simulink library "sensor_library"  (R2018b)
settings: Solver=VariableStepAuto  StartTime=0.0  StopTime=10.0  RelTol=1e-3
undefined symbols (not defined in the file): DiscIntNeverNeededParam, EOP_IERS, GPS, GPS_sensor_time, GYRO, GYRO_sensor_time, jdate0
libraries: dspsigops x26, simulink x9, simulink_extras x4
(part 1 of 2)
settings Model: Creator=Andrea  LastModifiedBy=andrea

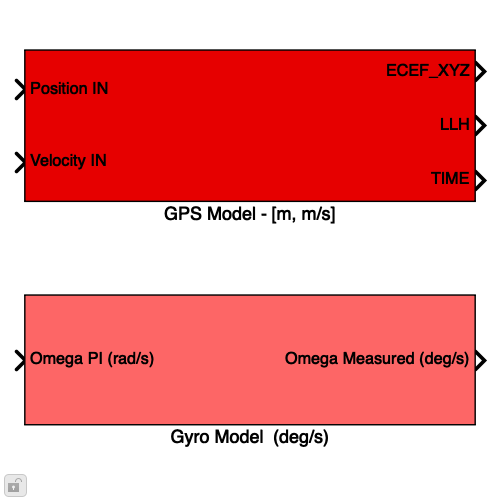
[thumbnail: Simulink's stored preview of the top-level diagram]
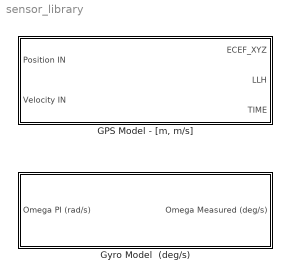
== system sensor_library ==
  "GPS Model - [m, m/s]" : Subsystem  mask{GPS=GPS, eop=EOP_IERS, jdutc_0=jdate0, simstep=GPS_sensor_time}
      mask prompts: GPS "GPS Data Structure"; eop "EOP (IERS) Parameter Structure"; jdutc_0 "Initial Simulation Time (UTC jdate)"; simstep "Sensor Time (s)"
  Gyro Model  (deg/s) : Subsystem  mask{gyros=GYRO.gyros, simstep=GYRO_sensor_time}
      mask prompts: gyros "Gyro Data Structure"; simstep "Sensor Time (s)"
      mask help:
      | Gyro Model - version A
      | Input - rad/s
      | Output - deg/s
      | Internal Data - deg/s

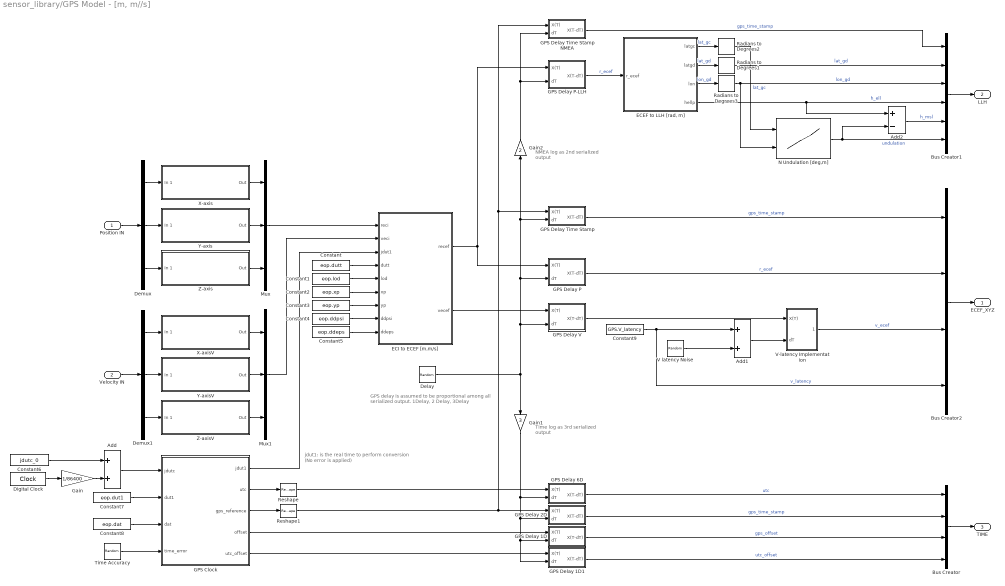
== system sensor_library/GPS Model - [m, m//s] ==
  note: NMEA log as 2nd
      | serialized output
  note: jdut1: is the real time to perform conversion
      | (No error is applied)
  note: GPS delay is assumed to be proportional among
      | all serialized output. 1Delay, 2 Delay, 3Delay
  note: Time log as 3rd
      | serialized output
  Position IN : Inport
  Velocity IN : Inport  Port=2
  Add : Sum
  Add1 : Sum
  Add2 : Sum  Inputs=+-
  Bus Creator : BusCreator  Inputs=4
  Bus Creator1 : BusCreator  Inputs=6
  Bus Creator2 : BusCreator  Inputs=4
  Constant : Constant  Value=eop.dutt  SampleTime=GPS.sampletime
  Constant1 : Constant  Value=eop.lod  SampleTime=GPS.sampletime
  Constant2 : Constant  Value=eop.xp  SampleTime=GPS.sampletime
  Constant3 : Constant  Value=eop.yp  SampleTime=GPS.sampletime
  Constant4 : Constant  Value=eop.ddpsi  SampleTime=GPS.sampletime
  Constant5 : Constant  Value=eop.ddeps  SampleTime=GPS.sampletime
  Constant6 : Constant  Value=jdutc_0  SampleTime=GPS.sampletime
  Constant7 : Constant  Value=eop.dut1  SampleTime=GPS.sampletime
  Constant8 : Constant  Value=eop.dat  SampleTime=GPS.sampletime
  Constant9 : Constant  Value=GPS.V_latency  SampleTime=GPS.sampletime
  Delay : RandomNumber  Mean=GPS.delay  Variance=GPS.delay_noise^2  Seed=GPS.noiseseedT-50  SampleTime=GPS.sampletime
  Demux : Demux  Outputs=3
  Demux1 : Demux  Outputs=3
  Digital Clock : DigitalClock  SampleTime=GPS.sampletime
  "ECEF to LLH [rad, m]" : MATLAB Function  TreatAsAtomicUnit=on
  ECI to ECEF [m,m/s] : MATLAB Function  TreatAsAtomicUnit=on
  GPS Clock : MATLAB Function  TreatAsAtomicUnit=on
  GPS Delay 1D : Subsystem  mask(Discrete Time Delay){maxT=1, Ts=GPS.sampletime}
      mask prompts: maxT "Max Delay Time (s)"; Ts "Sample Time (s)"
      mask help: Delay discrete-time input by a varying time, specified by the 'Delay' input dT, converted in fractional number of sample periods by means of indicated sample time. The input delay is clipped to a valid range (0 to dTMax) that is determined by the parameter settings. The block provides Linear interpolation modes.
  GPS Delay 1D1 : Subsystem  mask(Discrete Time Delay){maxT=1, Ts=GPS.sampletime}
      mask prompts: maxT "Max Delay Time (s)"; Ts "Sample Time (s)"
      mask help: Delay discrete-time input by a varying time, specified by the 'Delay' input dT, converted in fractional number of sample periods by means of indicated sample time. The input delay is clipped to a valid range (0 to dTMax) that is determined by the parameter settings. The block provides Linear interpolation modes.
  GPS Delay 2D : Subsystem  mask(Discrete Time Delay){maxT=1, Ts=GPS.sampletime}
      mask prompts: maxT "Max Delay Time (s)"; Ts "Sample Time (s)"
      mask help: Delay discrete-time input by a varying time, specified by the 'Delay' input dT, converted in fractional number of sample periods by means of indicated sample time. The input delay is clipped to a valid range (0 to dTMax) that is determined by the parameter settings. The block provides Linear interpolation modes.
  GPS Delay 6D : Subsystem  mask(Discrete Time Delay){maxT=1, Ts=GPS.sampletime}
      mask prompts: maxT "Max Delay Time (s)"; Ts "Sample Time (s)"
      mask help: Delay discrete-time input by a varying time, specified by the 'Delay' input dT, converted in fractional number of sample periods by means of indicated sample time. The input delay is clipped to a valid range (0 to dTMax) that is determined by the parameter settings. The block provides Linear interpolation modes.
  GPS Delay P : Subsystem  mask(Discrete Time Delay){maxT=1, Ts=GPS.sampletime}
      mask prompts: maxT "Max Delay Time (s)"; Ts "Sample Time (s)"
      mask help: Delay discrete-time input by a varying time, specified by the 'Delay' input dT, converted in fractional number of sample periods by means of indicated sample time. The input delay is clipped to a valid range (0 to dTMax) that is determined by the parameter settings. The block provides Linear interpolation modes.
  GPS Delay P-LLH : Subsystem  mask(Discrete Time Delay){maxT=1, Ts=GPS.sampletime}
      mask prompts: maxT "Max Delay Time (s)"; Ts "Sample Time (s)"
      mask help: Delay discrete-time input by a varying time, specified by the 'Delay' input dT, converted in fractional number of sample periods by means of indicated sample time. The input delay is clipped to a valid range (0 to dTMax) that is determined by the parameter settings. The block provides Linear interpolation modes.
  GPS Delay Time Stamp : Subsystem  mask(Discrete Time Delay){maxT=1, Ts=GPS.sampletime}
      mask prompts: maxT "Max Delay Time (s)"; Ts "Sample Time (s)"
      mask help: Delay discrete-time input by a varying time, specified by the 'Delay' input dT, converted in fractional number of sample periods by means of indicated sample time. The input delay is clipped to a valid range (0 to dTMax) that is determined by the parameter settings. The block provides Linear interpolation modes.
  GPS Delay Time Stamp NMEA : Subsystem  mask(Discrete Time Delay){maxT=1, Ts=GPS.sampletime}
      mask prompts: maxT "Max Delay Time (s)"; Ts "Sample Time (s)"
      mask help: Delay discrete-time input by a varying time, specified by the 'Delay' input dT, converted in fractional number of sample periods by means of indicated sample time. The input delay is clipped to a valid range (0 to dTMax) that is determined by the parameter settings. The block provides Linear interpolation modes.
  GPS Delay V : Subsystem  mask(Discrete Time Delay){maxT=1, Ts=GPS.sampletime}
      mask prompts: maxT "Max Delay Time (s)"; Ts "Sample Time (s)"
      mask help: Delay discrete-time input by a varying time, specified by the 'Delay' input dT, converted in fractional number of sample periods by means of indicated sample time. The input delay is clipped to a valid range (0 to dTMax) that is determined by the parameter settings. The block provides Linear interpolation modes.
  Gain : Gain  Gain=1/86400
  Gain1 : Gain  Gain=3
  Gain2 : Gain  Gain=2
  Mux : Mux  Inputs=3
  Mux1 : Mux  Inputs=3
  N Undulation [deg,m] : Lookup_n-D  BreakpointsForDimension1=[-90:1:90]  BreakpointsForDimension2=[-180:1:180]  Table=eop.N  InternalRulePriority=Speed  RndMeth=Simplest  InputSameDT=on
  Radians to Degrees1 : simulink_extras/Transformations/Radians to Degrees
  Radians to Degrees2 : simulink_extras/Transformations/Radians to Degrees
  Radians to Degrees3 : simulink_extras/Transformations/Radians to Degrees
  Reshape : Reshape
  Reshape1 : Reshape
  Time Accuracy : RandomNumber  Variance=GPS.noiseT^2  Seed=GPS.noiseseedT  SampleTime=GPS.sampletime
  V latency Noise : RandomNumber  Variance=GPS.V_latency_noise^2  Seed=GPS.noiseseedT+20  SampleTime=GPS.sampletime
  V-latency Implementation : Subsystem  mask(Discrete Time Delay){maxT=1, Ts=GPS.sampletime}
      mask prompts: maxT "Max Delay Time (s)"; Ts "Sample Time (s)"
      mask help: Delay discrete-time input by a varying time, specified by the 'Delay' input dT, converted in fractional number of sample periods by means of indicated sample time. The input delay is clipped to a valid range (0 to dTMax) that is determined by the parameter settings. The block provides Linear interpolation modes.
  X-axis : Subsystem  mask{bias=GPS.bias(1), noise=GPS.noise(1), noiseseed=GPS.noiseseed(1), resolution=GPS.resolution, sampletime=GPS.sampletime}
      mask prompts: bias "Bias (m)"; noise "Noise (m)"; noiseseed "Noise Seed"; resolution "Resolution (m)"; sampletime "Sample Time (s)"
  X-axisV : Subsystem  mask{bias=GPS.biasV(1), noise=GPS.noiseV(1), noiseseed=GPS.noiseseedV(1), resolution=GPS.resolutionV, sampletime=GPS.sampletime}
      mask prompts: bias "Bias (m/s)"; noise "Noise (m/s)"; noiseseed "Noise Seed"; resolution "Resolution (m/s)"; sampletime "Sample Time (s)"
  Y-axis : Subsystem  mask{bias=GPS.bias(2), noise=GPS.noise(2), noiseseed=GPS.noiseseed(2), resolution=GPS.resolution, sampletime=GPS.sampletime}
      mask prompts: bias "Bias (m)"; noise "Noise (m)"; noiseseed "Noise Seed"; resolution "Resolution (m)"; sampletime "Sample Time (s)"
  Y-axisV : Subsystem  mask{bias=GPS.biasV(2), noise=GPS.noiseV(2), noiseseed=GPS.noiseseedV(2), resolution=GPS.resolutionV, sampletime=GPS.sampletime}
      mask prompts: bias "Bias (m/s)"; noise "Noise (m/s)"; noiseseed "Noise Seed"; resolution "Resolution (m/s)"; sampletime "Sample Time (s)"
  Z-axis : Subsystem  mask{bias=GPS.bias(3), noise=GPS.noise(3), noiseseed=GPS.noiseseed(3), resolution=GPS.resolution, sampletime=GPS.sampletime}
      mask prompts: bias "Bias (m)"; noise "Noise (m)"; noiseseed "Noise Seed"; resolution "Resolution (m)"; sampletime "Sample Time (s)"
  Z-axisV : Subsystem  mask{bias=GPS.biasV(3), noise=GPS.noiseV(3), noiseseed=GPS.noiseseedV(3), resolution=GPS.resolutionV, sampletime=GPS.sampletime}
      mask prompts: bias "Bias (m/s)"; noise "Noise (m/s)"; noiseseed "Noise Seed"; resolution "Resolution (m/s)"; sampletime "Sample Time (s)"
  ECEF_XYZ : Outport  VectorParamsAs1DForOutWhenUnconnected=off
  LLH : Outport  Port=2  VectorParamsAs1DForOutWhenUnconnected=off
  TIME : Outport  Port=3  VectorParamsAs1DForOutWhenUnconnected=off
  wires:
  GPS Delay Time Stamp NMEA/1(X(T-dT)) -> Bus Creator1/1  "gps_time_stamp"
  Gain2/1 -> GPS Delay P-LLH/2(dT), GPS Delay Time Stamp NMEA/2(dT)
  Gain1/1 -> GPS Delay 1D1/2(dT), GPS Delay 1D/2(dT), GPS Delay 2D/2(dT), GPS Delay 6D/2(dT)
  GPS Delay Time Stamp/1(X(T-dT)) -> Bus Creator2/1  "gps_time_stamp"
  GPS Delay 1D1/1(X(T-dT)) -> Bus Creator/4  "utc_offset"
  GPS Clock/5(utc_offset) -> GPS Delay 1D1/1(X(T))
  GPS Delay 1D/1(X(T-dT)) -> Bus Creator/3  "gps_offset"
  GPS Clock/4(offset) -> GPS Delay 1D/1(X(T))
  GPS Delay 2D/1(X(T-dT)) -> Bus Creator/2  "gps_time_stamp"
  Reshape1/1 -> GPS Delay 2D/1(X(T)), GPS Delay Time Stamp/1(X(T)), GPS Delay Time Stamp NMEA/1(X(T))
  GPS Delay 6D/1(X(T-dT)) -> Bus Creator/1  "utc"
  Delay/1 -> Gain1/1, Gain2/1, GPS Delay Time Stamp/2(dT), GPS Delay P/2(dT), GPS Delay V/2(dT)
  GPS Delay P-LLH/1(X(T-dT)) -> "ECEF to LLH [rad, m]"/1(r_ecef)  "r_ecef"
  GPS Delay V/1(X(T-dT)) -> V-latency Implementation/1(X(T))
  GPS Delay P/1(X(T-dT)) -> Bus Creator2/2  "r_ecef"
  ECI to ECEF [m,m/s]/1(recef) -> GPS Delay P/1(X(T)), GPS Delay P-LLH/1(X(T))
  ECI to ECEF [m,m/s]/2(vecef) -> GPS Delay V/1(X(T))
  Add1/1 -> V-latency Implementation/2(dT)
  Constant9/1 -> Add1/1, Bus Creator2/4  "v_latency"
  Time Accuracy/1 -> GPS Clock/4(time_error)
  V-latency Implementation/1(X(T-dT)) -> Bus Creator2/3  "v_ecef"
  V latency Noise/1 -> Add1/2
  Digital Clock/1 -> Gain/1
  Reshape/1 -> GPS Delay 6D/1(X(T))
  Bus Creator2/1 -> ECEF_XYZ/1
  Bus Creator1/1 -> LLH/1
  Bus Creator/1 -> TIME/1
  Add2/1 -> Bus Creator1/5  "h_msl"
  N Undulation [deg,m]/1 -> Add2/2, Bus Creator1/6  "undulation"
  Radians to Degrees3/1 -> N Undulation [deg,m]/2, Bus Creator1/3  "lon_gd"
  Radians to Degrees2/1 -> N Undulation [deg,m]/1  "lat_gc"
  GPS Clock/3(gps_reference) -> Reshape1/1
  GPS Clock/2(utc) -> Reshape/1
  "ECEF to LLH [rad, m]"/4(hellp) -> Add2/1, Bus Creator1/4  "h_ell"
  "ECEF to LLH [rad, m]"/3(lon) -> Radians to Degrees3/1  "lon_gd"
  "ECEF to LLH [rad, m]"/2(latgd) -> Radians to Degrees1/1  "lat_gd"
  "ECEF to LLH [rad, m]"/1(latgc) -> Radians to Degrees2/1  "lat_gc"
  GPS Clock/1(jdut1) -> ECI to ECEF [m,m/s]/3(jdut1)
  Constant8/1 -> GPS Clock/3(dat)
  Constant7/1 -> GPS Clock/2(dut1)
  Add/1 -> GPS Clock/1(jdutc)
  Constant6/1 -> Add/1
  Gain/1 -> Add/2
  Constant5/1 -> ECI to ECEF [m,m/s]/9(ddeps)
  Constant4/1 -> ECI to ECEF [m,m/s]/8(ddpsi)
  Constant3/1 -> ECI to ECEF [m,m/s]/7(yp)
  Constant2/1 -> ECI to ECEF [m,m/s]/6(xp)
  Constant1/1 -> ECI to ECEF [m,m/s]/5(lod)
  Constant/1 -> ECI to ECEF [m,m/s]/4(dutt)
  Position IN/1 -> Demux/1
  Z-axis/1(Out) -> Mux/3
  Demux/3 -> Z-axis/1(In 1)
  Demux/1 -> X-axis/1(In 1)
  Y-axis/1(Out) -> Mux/2
  X-axis/1(Out) -> Mux/1
  Demux/2 -> Y-axis/1(In 1)
  Mux/1 -> ECI to ECEF [m,m/s]/1(reci)
  Mux1/1 -> ECI to ECEF [m,m/s]/2(veci)
  Demux1/2 -> Y-axisV/1(In 1)
  X-axisV/1(Out) -> Mux1/1
  Y-axisV/1(Out) -> Mux1/2
  Demux1/1 -> X-axisV/1(In 1)
  Demux1/3 -> Z-axisV/1(In 1)
  Z-axisV/1(Out) -> Mux1/3
  Velocity IN/1 -> Demux1/1
  Radians to Degrees1/1 -> Bus Creator1/2  "lat_gd"

== system sensor_library/Gyro Model  (deg//s) ==
  note: * Input Range Modelled
      | * Sample rate and Resolution Modelled
      | * Bias Modelled (Varying random at each start-up - Non-repeatability Modelled)
      | * Bias Instability Modelled
      | * Scale Factor Errors (Linear, Asymmetric, nonlinear) Modelled
      | * Sensor Noise (Random Walk and White Noise) Modelled
      | * Sensor non-orthogonality (Cross Axis Sensitivity) Modelled
      | * Latency Modelled
      | * Sensor mounting error (Small errors w.r.t. to nominal PI-IMU mounting) Modelled
      |
      | * Temperature effects NOT Modelled (Assumed T ~ const in S/C. Worst case scenario T to set initialization parameters)
      |
      | * G dependency and sensitivity NOT Modelled (Assumed G~0 in S/C. Included in the IMU signal processing/conditioning before output)
  Omega PI (rad/s) : Inport
  " GYRO measurements" : Subsystem  mask{gyro_Range=gyros.range, gyro_samplerate=gyros.samplerate, gyro_Bias=gyros.bias, gyro_SFE=gyros.SFE, gyro_SFA=gyros.SFA, gyro_SFN=gyros.SFN, gyro_BS=gyros.BS, gyro_Ctime=gyros.ctime, gyro_BSseed=gyros.BSseed, gyro_randomwalk=gyros.randomwalk, gyro_noise=gyros.noise, gyro_noiseseed=gyros.noiseseed, MAT_GYRO_CROSS=gyros.mismat, gyro_Res=gyros.resolution, DCM_GYRO_PI=gyros.mountmat, DCM_GYRO_ERR=gyros.mounterr}
      mask prompts: gyro_Range "Gyrometers Range (deg/s)"; gyro_samplerate "Gyrometers Sampling Rate (Hz)"; gyro_Bias "Gyrometers Bias (deg/s)"; gyro_SFE "Gyrometers SFE (ppm)"; gyro_SFA "Gyrometers SFA (ppm)"; gyro_SFN "Gyrometers SFN (ppm)"; gyro_BS "Gyrometers Bias Stability (deg/s)"; gyro_Ctime "Gyrometers BS Corr. Time (s)"; gyro_BSseed "Gyrometers BS Seed"; gyro_randomwalk "Gyrometers Random Walk (deg/s)"; gyro_noise "Gyrometers Noise (deg/s)"; gyro_noiseseed "Gyrometers Noise Seed"; MAT_GYRO_CROSS "Gyrometers Cross Axis Error"; gyro_Res "Gyrometers Resolution (deg/s)"; DCM_GYRO_PI "Body to Gyrometers Axes Rotation Matrix"; DCM_GYRO_ERR "Gyrometers Error Rotation Matrix"
  Omega Measured (deg/s) : Outport  VectorParamsAs1DForOutWhenUnconnected=off
  wires:
  " GYRO measurements"/1(Measurements (deg/s)) -> Omega Measured (deg/s)/1
  Omega PI (rad/s)/1 -> " GYRO measurements"/1(Angular rates (rad/s))

== system sensor_library/GPS Model - [m, m//s]/GPS Delay 1D ==
  X(T) : Inport
  dT : Inport  Port=2
  Variable Fractional Delay3 : dspsigops/Variable Fractional Delay  mode=OBSOLETE  modeActive=Linear  L=4  FarrowL=4  R=10  alpha=1  dmax=maxT/Ts  InputProcessing=Columns as channels (frame based)  ic=0  noDFT=off  fallbackFIR=Clip to the minimum value necessary for centered kernel  fallbackFarrow=Clip to the minimum value necessary for centered kernel  roundingMode=Zero  overflowMode=off
      settings: SourceProductBaseCode=DS
  n_sample : Gain  Gain=1/Ts
  X(T-dT) : Outport  VectorParamsAs1DForOutWhenUnconnected=off
  wires:
  n_sample/1 -> Variable Fractional Delay3/2
  dT/1 -> n_sample/1
  Variable Fractional Delay3/1 -> X(T-dT)/1
  X(T)/1 -> Variable Fractional Delay3/1

== system sensor_library/GPS Model - [m, m//s]/GPS Delay 1D1 ==
  X(T) : Inport
  dT : Inport  Port=2
  Variable Fractional Delay3 : dspsigops/Variable Fractional Delay  mode=OBSOLETE  modeActive=Linear  L=4  FarrowL=4  R=10  alpha=1  dmax=maxT/Ts  InputProcessing=Columns as channels (frame based)  ic=0  noDFT=off  fallbackFIR=Clip to the minimum value necessary for centered kernel  fallbackFarrow=Clip to the minimum value necessary for centered kernel  roundingMode=Zero  overflowMode=off
      settings: SourceProductBaseCode=DS
  n_sample : Gain  Gain=1/Ts
  X(T-dT) : Outport  VectorParamsAs1DForOutWhenUnconnected=off
  wires:
  X(T)/1 -> Variable Fractional Delay3/1
  Variable Fractional Delay3/1 -> X(T-dT)/1
  dT/1 -> n_sample/1
  n_sample/1 -> Variable Fractional Delay3/2

== system sensor_library/GPS Model - [m, m//s]/GPS Delay 2D ==
  X(T) : Inport
  dT : Inport  Port=2
  Demux : Demux  Outputs=2
  Mux : Mux  Inputs=2
  Variable Fractional Delay2 : dspsigops/Variable Fractional Delay  mode=OBSOLETE  modeActive=Linear  L=4  FarrowL=4  R=10  alpha=1  dmax=maxT/Ts  InputProcessing=Columns as channels (frame based)  ic=0  noDFT=off  fallbackFIR=Clip to the minimum value necessary for centered kernel  fallbackFarrow=Clip to the minimum value necessary for centered kernel  roundingMode=Zero  overflowMode=off
      settings: SourceProductBaseCode=DS
  Variable Fractional Delay3 : dspsigops/Variable Fractional Delay  mode=OBSOLETE  modeActive=Linear  L=4  FarrowL=4  R=10  alpha=1  dmax=maxT/Ts  InputProcessing=Columns as channels (frame based)  ic=0  noDFT=off  fallbackFIR=Clip to the minimum value necessary for centered kernel  fallbackFarrow=Clip to the minimum value necessary for centered kernel  roundingMode=Zero  overflowMode=off
      settings: SourceProductBaseCode=DS
  n_sample : Gain  Gain=1/Ts
  X(T-dT) : Outport  VectorParamsAs1DForOutWhenUnconnected=off
  wires:
  Variable Fractional Delay2/1 -> Mux/1
  Demux/2 -> Variable Fractional Delay3/1
  Demux/1 -> Variable Fractional Delay2/1
  Mux/1 -> X(T-dT)/1
  dT/1 -> n_sample/1
  X(T)/1 -> Demux/1
  n_sample/1 -> Variable Fractional Delay2/2, Variable Fractional Delay3/2
  Variable Fractional Delay3/1 -> Mux/2

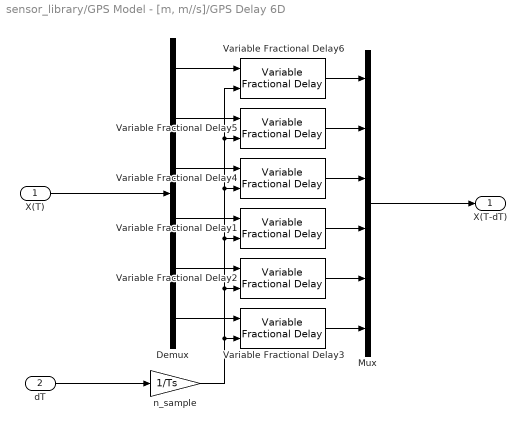
== system sensor_library/GPS Model - [m, m//s]/GPS Delay 6D ==
  X(T) : Inport
  dT : Inport  Port=2
  Demux : Demux  Outputs=6
  Mux : Mux  Inputs=6
  Variable Fractional Delay{1..6} (6 alike) : dspsigops/Variable Fractional Delay  mode=OBSOLETE  modeActive=Linear  L=4  FarrowL=4  R=10  alpha=1  dmax=maxT/Ts  InputProcessing=Columns as channels (frame based)  ic=0  noDFT=off  fallbackFIR=Clip to the minimum value necessary for centered kernel  fallbackFarrow=Clip to the minimum value necessary for centered kernel  roundingMode=Zero  overflowMode=off
      settings: SourceProductBaseCode=DS
  n_sample : Gain  Gain=1/Ts
  X(T-dT) : Outport  VectorParamsAs1DForOutWhenUnconnected=off
  wires:
  Variable Fractional Delay3/1 -> Mux/6
  Variable Fractional Delay2/1 -> Mux/5
  Variable Fractional Delay1/1 -> Mux/4
  Variable Fractional Delay4/1 -> Mux/3
  Variable Fractional Delay5/1 -> Mux/2
  Variable Fractional Delay6/1 -> Mux/1
  Demux/6 -> Variable Fractional Delay3/1
  Demux/5 -> Variable Fractional Delay2/1
  Demux/4 -> Variable Fractional Delay1/1
  Demux/3 -> Variable Fractional Delay4/1
  Demux/2 -> Variable Fractional Delay5/1
  Demux/1 -> Variable Fractional Delay6/1
  n_sample/1 -> Variable Fractional Delay3/2, Variable Fractional Delay2/2, Variable Fractional Delay1/2, Variable Fractional Delay4/2, Variable Fractional Delay5/2, Variable Fractional Delay6/2
  X(T)/1 -> Demux/1
  dT/1 -> n_sample/1
  Mux/1 -> X(T-dT)/1

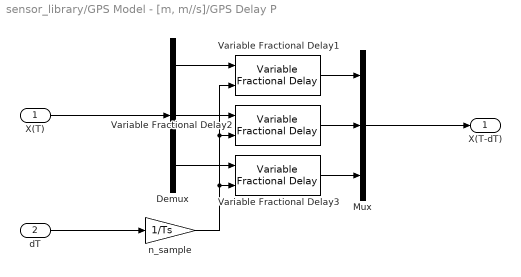
== system sensor_library/GPS Model - [m, m//s]/GPS Delay P ==
  X(T) : Inport
  dT : Inport  Port=2
  Demux : Demux  Outputs=3
  Mux : Mux  Inputs=3
  Variable Fractional Delay1 : dspsigops/Variable Fractional Delay  mode=OBSOLETE  modeActive=Linear  L=4  FarrowL=4  R=10  alpha=1  dmax=maxT/Ts  InputProcessing=Columns as channels (frame based)  ic=0  noDFT=off  fallbackFIR=Clip to the minimum value necessary for centered kernel  fallbackFarrow=Clip to the minimum value necessary for centered kernel  roundingMode=Zero  overflowMode=off
      settings: SourceProductBaseCode=DS
  Variable Fractional Delay2 : dspsigops/Variable Fractional Delay  mode=OBSOLETE  modeActive=Linear  L=4  FarrowL=4  R=10  alpha=1  dmax=maxT/Ts  InputProcessing=Columns as channels (frame based)  ic=0  noDFT=off  fallbackFIR=Clip to the minimum value necessary for centered kernel  fallbackFarrow=Clip to the minimum value necessary for centered kernel  roundingMode=Zero  overflowMode=off
      settings: SourceProductBaseCode=DS
  Variable Fractional Delay3 : dspsigops/Variable Fractional Delay  mode=OBSOLETE  modeActive=Linear  L=4  FarrowL=4  R=10  alpha=1  dmax=maxT/Ts  InputProcessing=Columns as channels (frame based)  ic=0  noDFT=off  fallbackFIR=Clip to the minimum value necessary for centered kernel  fallbackFarrow=Clip to the minimum value necessary for centered kernel  roundingMode=Zero  overflowMode=off
      settings: SourceProductBaseCode=DS
  n_sample : Gain  Gain=1/Ts
  X(T-dT) : Outport  VectorParamsAs1DForOutWhenUnconnected=off
  wires:
  Variable Fractional Delay1/1 -> Mux/1
  Mux/1 -> X(T-dT)/1
  dT/1 -> n_sample/1
  X(T)/1 -> Demux/1
  Demux/1 -> Variable Fractional Delay1/1
  Demux/3 -> Variable Fractional Delay3/1
  Variable Fractional Delay3/1 -> Mux/3
  Variable Fractional Delay2/1 -> Mux/2
  Demux/2 -> Variable Fractional Delay2/1
  n_sample/1 -> Variable Fractional Delay1/2, Variable Fractional Delay2/2, Variable Fractional Delay3/2

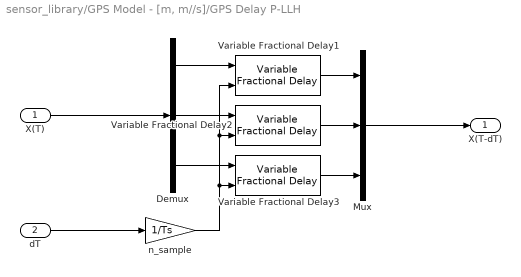
== system sensor_library/GPS Model - [m, m//s]/GPS Delay P-LLH ==
  X(T) : Inport
  dT : Inport  Port=2
  Demux : Demux  Outputs=3
  Mux : Mux  Inputs=3
  Variable Fractional Delay1 : dspsigops/Variable Fractional Delay  mode=OBSOLETE  modeActive=Linear  L=4  FarrowL=4  R=10  alpha=1  dmax=maxT/Ts  InputProcessing=Columns as channels (frame based)  ic=0  noDFT=off  fallbackFIR=Clip to the minimum value necessary for centered kernel  fallbackFarrow=Clip to the minimum value necessary for centered kernel  roundingMode=Zero  overflowMode=off
      settings: SourceProductBaseCode=DS
  Variable Fractional Delay2 : dspsigops/Variable Fractional Delay  mode=OBSOLETE  modeActive=Linear  L=4  FarrowL=4  R=10  alpha=1  dmax=maxT/Ts  InputProcessing=Columns as channels (frame based)  ic=0  noDFT=off  fallbackFIR=Clip to the minimum value necessary for centered kernel  fallbackFarrow=Clip to the minimum value necessary for centered kernel  roundingMode=Zero  overflowMode=off
      settings: SourceProductBaseCode=DS
  Variable Fractional Delay3 : dspsigops/Variable Fractional Delay  mode=OBSOLETE  modeActive=Linear  L=4  FarrowL=4  R=10  alpha=1  dmax=maxT/Ts  InputProcessing=Columns as channels (frame based)  ic=0  noDFT=off  fallbackFIR=Clip to the minimum value necessary for centered kernel  fallbackFarrow=Clip to the minimum value necessary for centered kernel  roundingMode=Zero  overflowMode=off
      settings: SourceProductBaseCode=DS
  n_sample : Gain  Gain=1/Ts
  X(T-dT) : Outport  VectorParamsAs1DForOutWhenUnconnected=off
  wires:
  n_sample/1 -> Variable Fractional Delay3/2, Variable Fractional Delay2/2, Variable Fractional Delay1/2
  Demux/2 -> Variable Fractional Delay2/1
  Variable Fractional Delay2/1 -> Mux/2
  Variable Fractional Delay3/1 -> Mux/3
  Demux/3 -> Variable Fractional Delay3/1
  Demux/1 -> Variable Fractional Delay1/1
  X(T)/1 -> Demux/1
  dT/1 -> n_sample/1
  Mux/1 -> X(T-dT)/1
  Variable Fractional Delay1/1 -> Mux/1

== system sensor_library/GPS Model - [m, m//s]/GPS Delay Time Stamp ==
  X(T) : Inport
  dT : Inport  Port=2
  Demux : Demux  Outputs=2
  Mux : Mux  Inputs=2
  Variable Fractional Delay2 : dspsigops/Variable Fractional Delay  mode=OBSOLETE  modeActive=Linear  L=4  FarrowL=4  R=10  alpha=1  dmax=maxT/Ts  InputProcessing=Columns as channels (frame based)  ic=0  noDFT=off  fallbackFIR=Clip to the minimum value necessary for centered kernel  fallbackFarrow=Clip to the minimum value necessary for centered kernel  roundingMode=Zero  overflowMode=off
      settings: SourceProductBaseCode=DS
  Variable Fractional Delay3 : dspsigops/Variable Fractional Delay  mode=OBSOLETE  modeActive=Linear  L=4  FarrowL=4  R=10  alpha=1  dmax=maxT/Ts  InputProcessing=Columns as channels (frame based)  ic=0  noDFT=off  fallbackFIR=Clip to the minimum value necessary for centered kernel  fallbackFarrow=Clip to the minimum value necessary for centered kernel  roundingMode=Zero  overflowMode=off
      settings: SourceProductBaseCode=DS
  n_sample : Gain  Gain=1/Ts
  X(T-dT) : Outport  VectorParamsAs1DForOutWhenUnconnected=off
  wires:
  Variable Fractional Delay3/1 -> Mux/2
  n_sample/1 -> Variable Fractional Delay3/2, Variable Fractional Delay2/2
  X(T)/1 -> Demux/1
  dT/1 -> n_sample/1
  Mux/1 -> X(T-dT)/1
  Demux/1 -> Variable Fractional Delay2/1
  Demux/2 -> Variable Fractional Delay3/1
  Variable Fractional Delay2/1 -> Mux/1

== system sensor_library/GPS Model - [m, m//s]/GPS Delay Time Stamp NMEA ==
  X(T) : Inport
  dT : Inport  Port=2
  Demux : Demux  Outputs=2
  Mux : Mux  Inputs=2
  Variable Fractional Delay2 : dspsigops/Variable Fractional Delay  mode=OBSOLETE  modeActive=Linear  L=4  FarrowL=4  R=10  alpha=1  dmax=maxT/Ts  InputProcessing=Columns as channels (frame based)  ic=0  noDFT=off  fallbackFIR=Clip to the minimum value necessary for centered kernel  fallbackFarrow=Clip to the minimum value necessary for centered kernel  roundingMode=Zero  overflowMode=off
      settings: SourceProductBaseCode=DS
  Variable Fractional Delay3 : dspsigops/Variable Fractional Delay  mode=OBSOLETE  modeActive=Linear  L=4  FarrowL=4  R=10  alpha=1  dmax=maxT/Ts  InputProcessing=Columns as channels (frame based)  ic=0  noDFT=off  fallbackFIR=Clip to the minimum value necessary for centered kernel  fallbackFarrow=Clip to the minimum value necessary for centered kernel  roundingMode=Zero  overflowMode=off
      settings: SourceProductBaseCode=DS
  n_sample : Gain  Gain=1/Ts
  X(T-dT) : Outport  VectorParamsAs1DForOutWhenUnconnected=off
  wires:
  Variable Fractional Delay3/1 -> Mux/2
  n_sample/1 -> Variable Fractional Delay3/2, Variable Fractional Delay2/2
  X(T)/1 -> Demux/1
  dT/1 -> n_sample/1
  Mux/1 -> X(T-dT)/1
  Demux/1 -> Variable Fractional Delay2/1
  Demux/2 -> Variable Fractional Delay3/1
  Variable Fractional Delay2/1 -> Mux/1

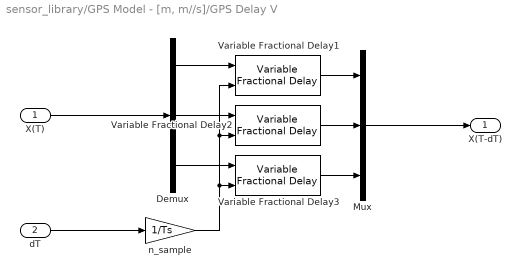
== system sensor_library/GPS Model - [m, m//s]/GPS Delay V ==
  X(T) : Inport
  dT : Inport  Port=2
  Demux : Demux  Outputs=3
  Mux : Mux  Inputs=3
  Variable Fractional Delay1 : dspsigops/Variable Fractional Delay  mode=OBSOLETE  modeActive=Linear  L=4  FarrowL=4  R=10  alpha=1  dmax=maxT/Ts  InputProcessing=Columns as channels (frame based)  ic=0  noDFT=off  fallbackFIR=Clip to the minimum value necessary for centered kernel  fallbackFarrow=Clip to the minimum value necessary for centered kernel  roundingMode=Zero  overflowMode=off
      settings: SourceProductBaseCode=DS
  Variable Fractional Delay2 : dspsigops/Variable Fractional Delay  mode=OBSOLETE  modeActive=Linear  L=4  FarrowL=4  R=10  alpha=1  dmax=maxT/Ts  InputProcessing=Columns as channels (frame based)  ic=0  noDFT=off  fallbackFIR=Clip to the minimum value necessary for centered kernel  fallbackFarrow=Clip to the minimum value necessary for centered kernel  roundingMode=Zero  overflowMode=off
      settings: SourceProductBaseCode=DS
  Variable Fractional Delay3 : dspsigops/Variable Fractional Delay  mode=OBSOLETE  modeActive=Linear  L=4  FarrowL=4  R=10  alpha=1  dmax=maxT/Ts  InputProcessing=Columns as channels (frame based)  ic=0  noDFT=off  fallbackFIR=Clip to the minimum value necessary for centered kernel  fallbackFarrow=Clip to the minimum value necessary for centered kernel  roundingMode=Zero  overflowMode=off
      settings: SourceProductBaseCode=DS
  n_sample : Gain  Gain=1/Ts
  X(T-dT) : Outport  VectorParamsAs1DForOutWhenUnconnected=off
  wires:
  n_sample/1 -> Variable Fractional Delay3/2, Variable Fractional Delay2/2, Variable Fractional Delay1/2
  Demux/2 -> Variable Fractional Delay2/1
  Variable Fractional Delay2/1 -> Mux/2
  Variable Fractional Delay3/1 -> Mux/3
  Demux/3 -> Variable Fractional Delay3/1
  Demux/1 -> Variable Fractional Delay1/1
  X(T)/1 -> Demux/1
  dT/1 -> n_sample/1
  Mux/1 -> X(T-dT)/1
  Variable Fractional Delay1/1 -> Mux/1

== system sensor_library/GPS Model - [m, m//s]/V-latency Implementation ==
  X(T) : Inport
  dT : Inport  Port=2
  Demux : Demux  Outputs=3
  Mux : Mux  Inputs=3
  Variable Fractional Delay1 : dspsigops/Variable Fractional Delay  mode=OBSOLETE  modeActive=Linear  L=4  FarrowL=4  R=10  alpha=1  dmax=maxT/Ts  InputProcessing=Columns as channels (frame based)  ic=0  noDFT=off  fallbackFIR=Clip to the minimum value necessary for centered kernel  fallbackFarrow=Clip to the minimum value necessary for centered kernel  roundingMode=Zero  overflowMode=off
      settings: SourceProductBaseCode=DS
  Variable Fractional Delay2 : dspsigops/Variable Fractional Delay  mode=OBSOLETE  modeActive=Linear  L=4  FarrowL=4  R=10  alpha=1  dmax=maxT/Ts  InputProcessing=Columns as channels (frame based)  ic=0  noDFT=off  fallbackFIR=Clip to the minimum value necessary for centered kernel  fallbackFarrow=Clip to the minimum value necessary for centered kernel  roundingMode=Zero  overflowMode=off
      settings: SourceProductBaseCode=DS
  Variable Fractional Delay3 : dspsigops/Variable Fractional Delay  mode=OBSOLETE  modeActive=Linear  L=4  FarrowL=4  R=10  alpha=1  dmax=maxT/Ts  InputProcessing=Columns as channels (frame based)  ic=0  noDFT=off  fallbackFIR=Clip to the minimum value necessary for centered kernel  fallbackFarrow=Clip to the minimum value necessary for centered kernel  roundingMode=Zero  overflowMode=off
      settings: SourceProductBaseCode=DS
  n_sample : Gain  Gain=1/Ts
  X(T-dT) : Outport  VectorParamsAs1DForOutWhenUnconnected=off
  wires:
  Variable Fractional Delay1/1 -> Mux/1
  Mux/1 -> X(T-dT)/1
  dT/1 -> n_sample/1
  X(T)/1 -> Demux/1
  Demux/1 -> Variable Fractional Delay1/1
  Demux/3 -> Variable Fractional Delay3/1
  Variable Fractional Delay3/1 -> Mux/3
  Variable Fractional Delay2/1 -> Mux/2
  Demux/2 -> Variable Fractional Delay2/1
  n_sample/1 -> Variable Fractional Delay1/2, Variable Fractional Delay2/2, Variable Fractional Delay3/2

== system sensor_library/GPS Model - [m, m//s]/X-axis ==
  note: On-axis signal
  In 1 : Inport
  ADC Quantizer : Quantizer  QuantizationInterval=resolution
  Fixed Bias / Bias Repeatability : Constant  Value=bias
  Random Number : RandomNumber  Variance=noise^2  Seed=noiseseed  SampleTime=sampletime
  Sum : Sum  Inputs=+++
  Zero-Order Hold : ZeroOrderHold  SampleTime=sampletime
  Out : Outport  VectorParamsAs1DForOutWhenUnconnected=off
  wires:
  Random Number/1 -> Sum/2
  In 1/1 -> Sum/1
  Sum/1 -> ADC Quantizer/1
  ADC Quantizer/1 -> Zero-Order Hold/1
  Zero-Order Hold/1 -> Out/1
  Fixed Bias / Bias Repeatability/1 -> Sum/3

== system sensor_library/GPS Model - [m, m//s]/X-axisV ==
  note: On-axis signal
  In 1 : Inport
  ADC Quantizer : Quantizer  QuantizationInterval=resolution
  Fixed Bias / Bias Repeatability : Constant  Value=bias
  Random Number : RandomNumber  Variance=noise^2  Seed=noiseseed  SampleTime=sampletime
  Sum : Sum  Inputs=+++
  Zero-Order Hold : ZeroOrderHold  SampleTime=sampletime
  Out : Outport  VectorParamsAs1DForOutWhenUnconnected=off
  wires:
  Fixed Bias / Bias Repeatability/1 -> Sum/3
  Zero-Order Hold/1 -> Out/1
  ADC Quantizer/1 -> Zero-Order Hold/1
  Sum/1 -> ADC Quantizer/1
  In 1/1 -> Sum/1
  Random Number/1 -> Sum/2

== system sensor_library/GPS Model - [m, m//s]/Y-axis ==
  note: On-axis signal
  In 1 : Inport
  ADC Quantizer : Quantizer  QuantizationInterval=resolution
  Fixed Bias / Bias Repeatability : Constant  Value=bias
  Random Number : RandomNumber  Variance=noise^2  Seed=noiseseed  SampleTime=sampletime
  Sum : Sum  Inputs=+++
  Zero-Order Hold : ZeroOrderHold  SampleTime=sampletime
  Out : Outport  VectorParamsAs1DForOutWhenUnconnected=off
  wires:
  Fixed Bias / Bias Repeatability/1 -> Sum/3
  Zero-Order Hold/1 -> Out/1
  ADC Quantizer/1 -> Zero-Order Hold/1
  Sum/1 -> ADC Quantizer/1
  In 1/1 -> Sum/1
  Random Number/1 -> Sum/2

== system sensor_library/GPS Model - [m, m//s]/Y-axisV ==
  note: On-axis signal
  In 1 : Inport
  ADC Quantizer : Quantizer  QuantizationInterval=resolution
  Fixed Bias / Bias Repeatability : Constant  Value=bias
  Random Number : RandomNumber  Variance=noise^2  Seed=noiseseed  SampleTime=sampletime
  Sum : Sum  Inputs=+++
  Zero-Order Hold : ZeroOrderHold  SampleTime=sampletime
  Out : Outport  VectorParamsAs1DForOutWhenUnconnected=off
  wires:
  Random Number/1 -> Sum/2
  In 1/1 -> Sum/1
  Sum/1 -> ADC Quantizer/1
  ADC Quantizer/1 -> Zero-Order Hold/1
  Zero-Order Hold/1 -> Out/1
  Fixed Bias / Bias Repeatability/1 -> Sum/3

== system sensor_library/GPS Model - [m, m//s]/Z-axis ==
  note: On-axis signal
  In 1 : Inport
  ADC Quantizer : Quantizer  QuantizationInterval=resolution
  Fixed Bias / Bias Repeatability : Constant  Value=bias
  Random Number : RandomNumber  Variance=noise^2  Seed=noiseseed  SampleTime=sampletime
  Sum : Sum  Inputs=+++
  Zero-Order Hold : ZeroOrderHold  SampleTime=sampletime
  Out : Outport  VectorParamsAs1DForOutWhenUnconnected=off
  wires:
  Random Number/1 -> Sum/2
  In 1/1 -> Sum/1
  Sum/1 -> ADC Quantizer/1
  ADC Quantizer/1 -> Zero-Order Hold/1
  Zero-Order Hold/1 -> Out/1
  Fixed Bias / Bias Repeatability/1 -> Sum/3

== system sensor_library/GPS Model - [m, m//s]/Z-axisV ==
  note: On-axis signal
  In 1 : Inport
  ADC Quantizer : Quantizer  QuantizationInterval=resolution
  Fixed Bias / Bias Repeatability : Constant  Value=bias
  Random Number : RandomNumber  Variance=noise^2  Seed=noiseseed  SampleTime=sampletime
  Sum : Sum  Inputs=+++
  Zero-Order Hold : ZeroOrderHold  SampleTime=sampletime
  Out : Outport  VectorParamsAs1DForOutWhenUnconnected=off
  wires:
  Fixed Bias / Bias Repeatability/1 -> Sum/3
  Zero-Order Hold/1 -> Out/1
  ADC Quantizer/1 -> Zero-Order Hold/1
  Sum/1 -> ADC Quantizer/1
  In 1/1 -> Sum/1
  Random Number/1 -> Sum/2

== system sensor_library/Gyro Model  (deg//s)/ GYRO measurements ==
  Angular rates (rad/s) : Inport
  Gyros Triad : Subsystem  mask{samplerate=gyro_samplerate}
      mask prompts: samplerate "Gyro Sampling Rate (Hz)"
  Mounting Body to GYRO : Product  Multiplication=Matrix(*)  RndMeth=Zero
  Mounting Error : Product  Multiplication=Matrix(*)  RndMeth=Zero
  Radians to Degrees : simulink_extras/Transformations/Radians to Degrees
  wl_ins1 : Constant  Value=DCM_GYRO_ERR
  wl_ins2 : Constant  Value=DCM_GYRO_PI
  Measurements (deg/s) : Outport  VectorParamsAs1DForOutWhenUnconnected=off
  wires:
  Angular rates (rad/s)/1 -> Mounting Body to GYRO/2
  Radians to Degrees/1 -> Gyros Triad/1(In1)
  Gyros Triad/1(Out1) -> Measurements (deg/s)/1
  wl_ins2/1 -> Mounting Error/2
  Mounting Body to GYRO/1 -> Radians to Degrees/1
  Mounting Error/1 -> Mounting Body to GYRO/1
  wl_ins1/1 -> Mounting Error/1

== system sensor_library/Gyro Model  (deg//s)/ GYRO measurements/Gyros Triad ==
  In1 : Inport
  Cross Axis : Product  Multiplication=Matrix(*)  RndMeth=Zero
  Demux : Demux  Outputs=3
  Mux : Mux  Inputs=3
  X-axis Gyro : Subsystem  mask{range=gyro_Range(1), SFE=gyro_SFE(1), SFA=gyro_SFA(1), SFN=gyro_SFN(1), bias=gyro_Bias(1), noise=gyro_noise(1), BS=gyro_BS(1), random_walk=gyro_randomwalk(1), ctime=gyro_Ctime(1), resolution=gyro_Res(1), noiseseed=gyro_noiseseed(1), BSseed=gyro_BSseed(1)}
      mask prompts: range "Range (deg/s)"; SFE "Scale Factor Error (ppm)"; SFA "Scale Factor Asimmetry (ppm)"; SFN "Scale Factor Nonlinearity (ppm)"; bias "Bias Repeatability (deg/s)"; noise "White Noise (deg/s)"; BS "Bias Stability (deg/s)"; random_walk "Random Walk (deg/s)"; ctime "Correlation Time (s)"; resolution "Resolution (deg/s)"; noiseseed "Noise Seed"; BSseed "BS Seed"
  Y-axis Gyro : Subsystem  mask{range=gyro_Range(2), SFE=gyro_SFE(2), SFA=gyro_SFA(2), SFN=gyro_SFN(2), bias=gyro_Bias(2), noise=gyro_noise(2), BS=gyro_BS(2), random_walk=gyro_randomwalk(2), ctime=gyro_Ctime(2), resolution=gyro_Res(2), noiseseed=gyro_noiseseed(2), BSseed=gyro_BSseed(2)}
      mask prompts: range "Range (deg/s)"; SFE "Scale Factor Error (ppm)"; SFA "Scale Factor Asimmetry (ppm)"; SFN "Scale Factor Nonlinearity (ppm)"; bias "Bias Repeatability (deg/s)"; noise "White Noise (deg/s)"; BS "Bias Stability (deg/s)"; random_walk "Random Walk (deg/s)"; ctime "Correlation Time (s)"; resolution "Resolution (deg/s)"; noiseseed "Noise Seed"; BSseed "BS Seed"
  Z-axis Gyro : Subsystem  mask{range=gyro_Range(3), SFE=gyro_SFE(3), SFA=gyro_SFA(3), SFN=gyro_SFN(3), bias=gyro_Bias(3), noise=gyro_noise(3), BS=gyro_BS(3), random_walk=gyro_randomwalk(3), ctime=gyro_Ctime(3), resolution=gyro_Res(3), noiseseed=gyro_noiseseed(3), BSseed=gyro_BSseed(3)}
      mask prompts: range "Range (deg/s)"; SFE "Scale Factor Error (ppm)"; SFA "Scale Factor Asimmetry (ppm)"; SFN "Scale Factor Nonlinearity (ppm)"; bias "Bias Repeatability (deg/s)"; noise "White Noise (deg/s)"; BS "Bias Stability (deg/s)"; random_walk "Random Walk (deg/s)"; ctime "Correlation Time (s)"; resolution "Resolution (deg/s)"; noiseseed "Noise Seed"; BSseed "BS Seed"
  wl_ins1 : Constant  Value=MAT_GYRO_CROSS
  Out1 : Outport  VectorParamsAs1DForOutWhenUnconnected=off
  wires:
  wl_ins1/1 -> Cross Axis/1
  Cross Axis/1 -> Demux/1
  Y-axis Gyro/1(Out) -> Mux/2
  Z-axis Gyro/1(Out) -> Mux/3
  Demux/3 -> Z-axis Gyro/1(In)
  Demux/2 -> Y-axis Gyro/1(In)
  Demux/1 -> X-axis Gyro/1(In)
  In1/1 -> Cross Axis/2
  Mux/1 -> Out1/1
  X-axis Gyro/1(Out) -> Mux/1

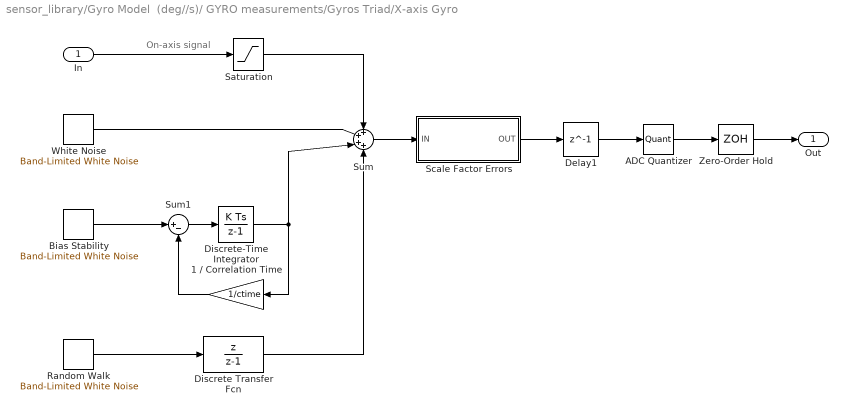
== system sensor_library/Gyro Model  (deg//s)/ GYRO measurements/Gyros Triad/X-axis Gyro ==
  note: On-axis signal
  In : Inport
  1 / Correlation Time : Gain  Gain=1/ctime
  ADC Quantizer : Quantizer  QuantizationInterval=resolution
  Bias Stability : simulink/Sources/Band-Limited White Noise  Cov=(2*(BS)^2)/ctime  Ts=simstep  seed=BSseed
  Delay1 : Delay  DelayLength=1  InitialCondition=0  SampleTime=1/samplerate
  Discrete Transfer Fcn : DiscreteTransferFcn  Numerator=[1 0]  Denominator=[1 -1]
  Discrete-Time Integrator : DiscreteIntegrator  SampleTime=1/samplerate  ICPrevOutput=DiscIntNeverNeededParam  ICPrevScaledInput=DiscIntNeverNeededParam
  Random Walk : simulink/Sources/Band-Limited White Noise  Cov=(random_walk*simstep)^2  Ts=simstep  seed=noiseseed*BSseed
  Saturation : Saturate  UpperLimit=range  LowerLimit=-range
  Scale Factor Errors : Subsystem
  Sum : Sum  Inputs=++++
  Sum1 : Sum  Inputs=|+-
  White Noise : simulink/Sources/Band-Limited White Noise  Cov=noise^2  Ts=simstep  seed=noiseseed
  Zero-Order Hold : ZeroOrderHold  SampleTime=1/samplerate
  Out : Outport  VectorParamsAs1DForOutWhenUnconnected=off
  wires:
  Random Walk/1 -> Discrete Transfer Fcn/1
  Discrete Transfer Fcn/1 -> Sum/4
  White Noise/1 -> Sum/2
  Zero-Order Hold/1 -> Out/1
  1 / Correlation Time/1 -> Sum1/2
  Scale Factor Errors/1(OUT) -> Delay1/1
  Delay1/1 -> ADC Quantizer/1
  ADC Quantizer/1 -> Zero-Order Hold/1
  Saturation/1 -> Sum/1
  In/1 -> Saturation/1
  Sum/1 -> Scale Factor Errors/1(IN)
  Discrete-Time Integrator/1 -> Sum/3, 1 / Correlation Time/1
  Sum1/1 -> Discrete-Time Integrator/1
  Bias Stability/1 -> Sum1/1

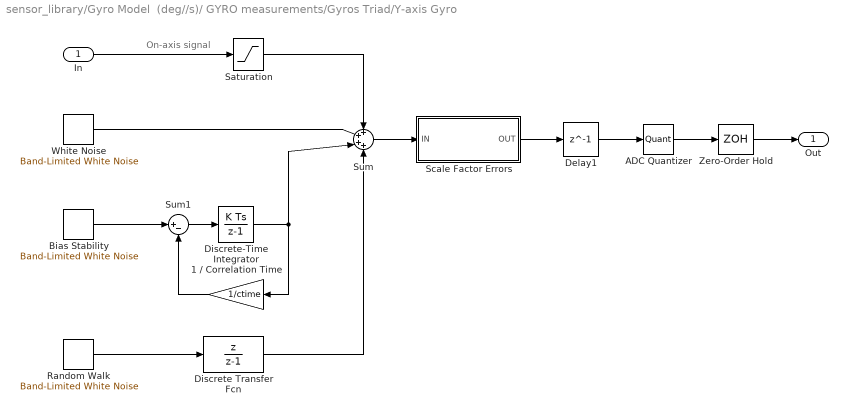
== system sensor_library/Gyro Model  (deg//s)/ GYRO measurements/Gyros Triad/Y-axis Gyro ==
  note: On-axis signal
  In : Inport
  1 / Correlation Time : Gain  Gain=1/ctime
  ADC Quantizer : Quantizer  QuantizationInterval=resolution
  Bias Stability : simulink/Sources/Band-Limited White Noise  Cov=(2*(BS)^2)/ctime  Ts=simstep  seed=BSseed
  Delay1 : Delay  DelayLength=1  InitialCondition=0  SampleTime=1/samplerate
  Discrete Transfer Fcn : DiscreteTransferFcn  Numerator=[1 0]  Denominator=[1 -1]
  Discrete-Time Integrator : DiscreteIntegrator  SampleTime=1/samplerate  ICPrevOutput=DiscIntNeverNeededParam  ICPrevScaledInput=DiscIntNeverNeededParam
  Random Walk : simulink/Sources/Band-Limited White Noise  Cov=(random_walk*simstep)^2  Ts=simstep  seed=noiseseed*BSseed
  Saturation : Saturate  UpperLimit=range  LowerLimit=-range
  Scale Factor Errors : Subsystem
  Sum : Sum  Inputs=++++
  Sum1 : Sum  Inputs=|+-
  White Noise : simulink/Sources/Band-Limited White Noise  Cov=noise^2  Ts=simstep  seed=noiseseed
  Zero-Order Hold : ZeroOrderHold  SampleTime=1/samplerate
  Out : Outport  VectorParamsAs1DForOutWhenUnconnected=off
  wires:
  Bias Stability/1 -> Sum1/1
  Sum1/1 -> Discrete-Time Integrator/1
  Discrete-Time Integrator/1 -> 1 / Correlation Time/1, Sum/3
  Sum/1 -> Scale Factor Errors/1(IN)
  In/1 -> Saturation/1
  Saturation/1 -> Sum/1
  ADC Quantizer/1 -> Zero-Order Hold/1
  Delay1/1 -> ADC Quantizer/1
  Scale Factor Errors/1(OUT) -> Delay1/1
  1 / Correlation Time/1 -> Sum1/2
  Zero-Order Hold/1 -> Out/1
  White Noise/1 -> Sum/2
  Discrete Transfer Fcn/1 -> Sum/4
  Random Walk/1 -> Discrete Transfer Fcn/1

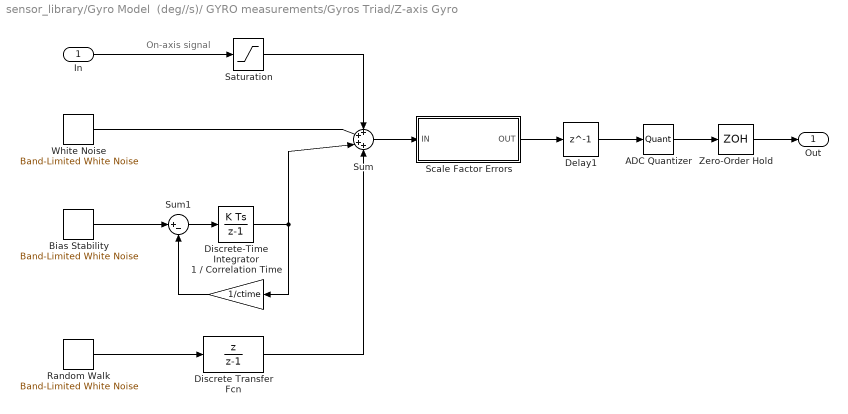
== system sensor_library/Gyro Model  (deg//s)/ GYRO measurements/Gyros Triad/Z-axis Gyro ==
  note: On-axis signal
  In : Inport
  1 / Correlation Time : Gain  Gain=1/ctime
  ADC Quantizer : Quantizer  QuantizationInterval=resolution
  Bias Stability : simulink/Sources/Band-Limited White Noise  Cov=(2*(BS)^2)/ctime  Ts=simstep  seed=BSseed
  Delay1 : Delay  DelayLength=1  InitialCondition=0  SampleTime=1/samplerate
  Discrete Transfer Fcn : DiscreteTransferFcn  Numerator=[1 0]  Denominator=[1 -1]
  Discrete-Time Integrator : DiscreteIntegrator  SampleTime=1/samplerate  ICPrevOutput=DiscIntNeverNeededParam  ICPrevScaledInput=DiscIntNeverNeededParam
  Random Walk : simulink/Sources/Band-Limited White Noise  Cov=(random_walk*simstep)^2  Ts=simstep  seed=noiseseed*BSseed
  Saturation : Saturate  UpperLimit=range  LowerLimit=-range
  Scale Factor Errors : Subsystem
  Sum : Sum  Inputs=++++
  Sum1 : Sum  Inputs=|+-
  White Noise : simulink/Sources/Band-Limited White Noise  Cov=noise^2  Ts=simstep  seed=noiseseed
  Zero-Order Hold : ZeroOrderHold  SampleTime=1/samplerate
  Out : Outport  VectorParamsAs1DForOutWhenUnconnected=off
  wires:
  Random Walk/1 -> Discrete Transfer Fcn/1
  Discrete Transfer Fcn/1 -> Sum/4
  White Noise/1 -> Sum/2
  Zero-Order Hold/1 -> Out/1
  1 / Correlation Time/1 -> Sum1/2
  Scale Factor Errors/1(OUT) -> Delay1/1
  Delay1/1 -> ADC Quantizer/1
  ADC Quantizer/1 -> Zero-Order Hold/1
  Saturation/1 -> Sum/1
  In/1 -> Saturation/1
  Sum/1 -> Scale Factor Errors/1(IN)
  Discrete-Time Integrator/1 -> Sum/3, 1 / Correlation Time/1
  Sum1/1 -> Discrete-Time Integrator/1
  Bias Stability/1 -> Sum1/1

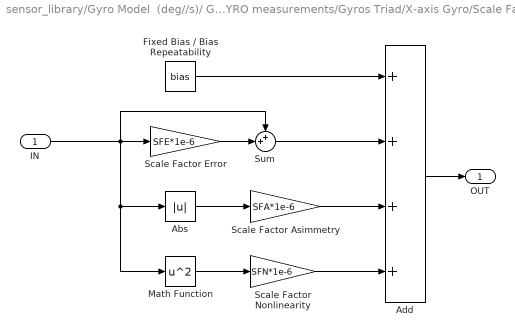
== system sensor_library/Gyro Model  (deg//s)/ GYRO measurements/Gyros Triad/X-axis Gyro/Scale Factor Errors ==
  IN : Inport
  Abs : Abs
  Add : Sum  Inputs=++++
  Fixed Bias / Bias Repeatability : Constant  Value=bias
  Math Function : Math  Operator=square  SaturateOnIntegerOverflow=on
  Scale Factor Asimmetry : Gain  Gain=SFA*1e-6
  Scale Factor Error : Gain  Gain=SFE*1e-6
  Scale Factor Nonlinearity : Gain  Gain=SFN*1e-6
  Sum : Sum  Inputs=++|
  OUT : Outport  VectorParamsAs1DForOutWhenUnconnected=off
  wires:
  Abs/1 -> Scale Factor Asimmetry/1
  Math Function/1 -> Scale Factor Nonlinearity/1
  Sum/1 -> Add/2
  Scale Factor Error/1 -> Sum/2
  Scale Factor Nonlinearity/1 -> Add/4
  Scale Factor Asimmetry/1 -> Add/3
  IN/1 -> Sum/1, Abs/1, Math Function/1, Scale Factor Error/1
  Fixed Bias / Bias Repeatability/1 -> Add/1
  Add/1 -> OUT/1

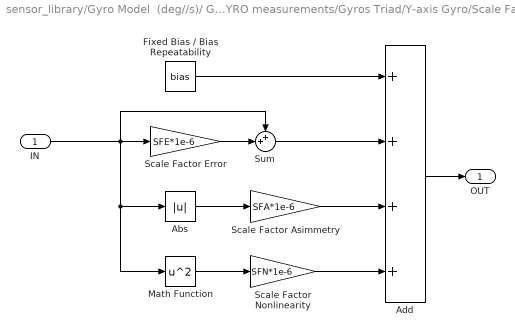
== system sensor_library/Gyro Model  (deg//s)/ GYRO measurements/Gyros Triad/Y-axis Gyro/Scale Factor Errors ==
  IN : Inport
  Abs : Abs
  Add : Sum  Inputs=++++
  Fixed Bias / Bias Repeatability : Constant  Value=bias
  Math Function : Math  Operator=square  SaturateOnIntegerOverflow=on
  Scale Factor Asimmetry : Gain  Gain=SFA*1e-6
  Scale Factor Error : Gain  Gain=SFE*1e-6
  Scale Factor Nonlinearity : Gain  Gain=SFN*1e-6
  Sum : Sum  Inputs=++|
  OUT : Outport  VectorParamsAs1DForOutWhenUnconnected=off
  wires:
  Add/1 -> OUT/1
  Fixed Bias / Bias Repeatability/1 -> Add/1
  IN/1 -> Scale Factor Error/1, Math Function/1, Abs/1, Sum/1
  Scale Factor Asimmetry/1 -> Add/3
  Scale Factor Nonlinearity/1 -> Add/4
  Scale Factor Error/1 -> Sum/2
  Sum/1 -> Add/2
  Math Function/1 -> Scale Factor Nonlinearity/1
  Abs/1 -> Scale Factor Asimmetry/1

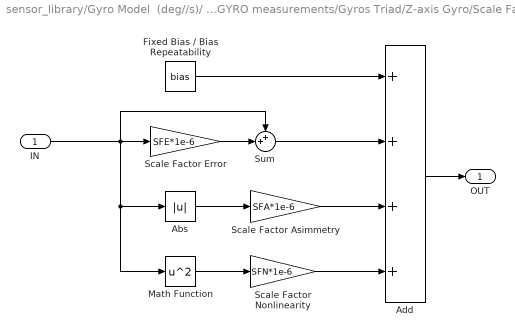
== system sensor_library/Gyro Model  (deg//s)/ GYRO measurements/Gyros Triad/Z-axis Gyro/Scale Factor Errors ==
  IN : Inport
  Abs : Abs
  Add : Sum  Inputs=++++
  Fixed Bias / Bias Repeatability : Constant  Value=bias
  Math Function : Math  Operator=square  SaturateOnIntegerOverflow=on
  Scale Factor Asimmetry : Gain  Gain=SFA*1e-6
  Scale Factor Error : Gain  Gain=SFE*1e-6
  Scale Factor Nonlinearity : Gain  Gain=SFN*1e-6
  Sum : Sum  Inputs=++|
  OUT : Outport  VectorParamsAs1DForOutWhenUnconnected=off
  wires:
  Abs/1 -> Scale Factor Asimmetry/1
  Math Function/1 -> Scale Factor Nonlinearity/1
  Sum/1 -> Add/2
  Scale Factor Error/1 -> Sum/2
  Scale Factor Nonlinearity/1 -> Add/4
  Scale Factor Asimmetry/1 -> Add/3
  IN/1 -> Sum/1, Abs/1, Math Function/1, Scale Factor Error/1
  Fixed Bias / Bias Repeatability/1 -> Add/1
  Add/1 -> OUT/1
